simulink model "Vectors"  (R2020a)
settings: Solver=VariableStepAuto  StartTime=0.0  StopTime=2  RelTol=1e-3
settings Model: Creator=ashok  LastModifiedBy=ashok

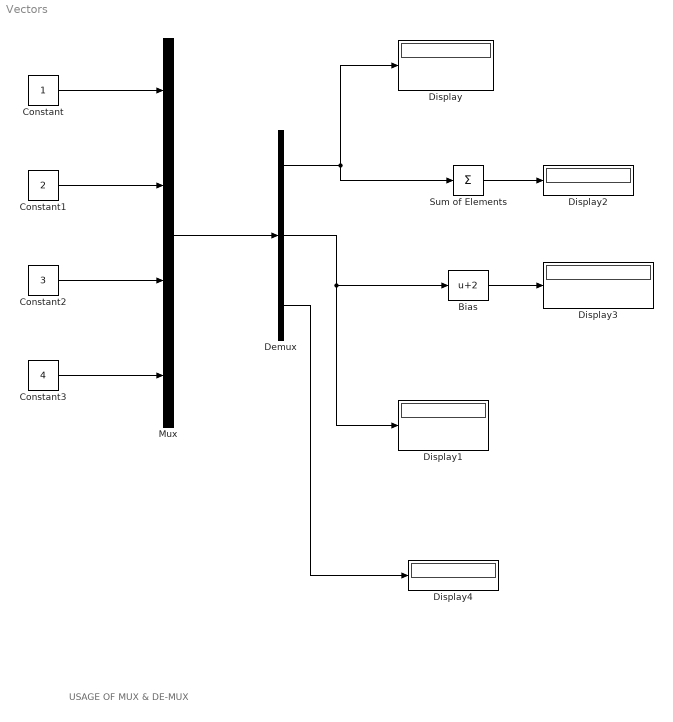
== system Vectors ==
  note: USAGE OF MUX & DE-MUX
  Bias : Bias  Bias=2
  Constant : Constant
  Constant1 : Constant  Value=2
  Constant2 : Constant  Value=3
  Constant3 : Constant  Value=4
  Demux : Demux  Outputs=3
  Display{,1..4} (5 alike) : Display
  Mux : Mux
  Sum of Elements : Sum  Inputs=+
  wires:
  Constant/1 -> Mux/1
  Constant1/1 -> Mux/2
  Constant2/1 -> Mux/3
  Constant3/1 -> Mux/4
  Mux/1 -> Demux/1
  Demux/1 -> Sum of Elements/1, Display/1
  Demux/2 -> Display1/1, Bias/1
  Sum of Elements/1 -> Display2/1
  Bias/1 -> Display3/1
  Demux/3 -> Display4/1
